simulink model "Vehicle_Model_contABS"  (R2022b)
settings: Solver=ode2  StartTime=T0  StopTime=Tf  FixedStep=Ts  EnableMultiTasking=on
model workspace (MAT data in the model file):
  aKalman = Simulink.Parameter
  aKalman.DataType = 'auto'
  aKalman.Complexity = 'real'
  aKalman.Dimensions = [0 0]
  slipEnabler = Simulink.Parameter
  slipEnabler.DataType = 'auto'
  slipEnabler.Complexity = 'real'
  slipEnabler.Dimensions = [0 0]
values from neighbouring files (symbols this model uses):
  enable_onlinePlots = 0    [main.m]
  enable_zoom = 1    [main.m]
  hv = 0.2    [main.m]
  lambda1_th = 0.1    [main.m]
  lambda2_th = 0.1    [main.m]
  LLC_sampleTime = LLC.sample_time    [main.m]
  longCTRparam = longitController()    [main.m]
  low_level_control = scenario_data.vehicle_control.low_level_control    [main.m]
  omega_LPF = 100    [main.m]
  previewPointParams = previewPointControllerParams()    [main.m]
  rho = 0.97    [main.m]
  rho_off = 0.9    [main.m]
  rho_on = 1.02    [main.m]
  road_data_sampled = [scenario_data.path.x_sampled', scenario_data.path.y_sampled']    [main.m]
  T0 = scenario_data.times.t0    [main.m]
  tau_delta = vehicle_data.steering_system.tau_D    [main.m]
  Tb_dot_max = 5e3    (= 5000)    [main.m]
  Tb_max = 3500    [main.m]
  Tf = scenario_data.times.tf    [main.m]
  Ts = scenario_data.times.step_size    [main.m]
  v_on = 2.5    [main.m]
  v_stop = 0.1    [main.m]
  vehicle_data = getVehicleDataStruct()    [main.m]
  X0 = loadInitialConditions(scenario_data.vehicle_control.max_speed/3.6)    [main.m]
undefined symbols (not defined in the file or in its folder): DiscIntNeverNeededParam, latContr_select
libraries: simulink_extras x20, simulink x9, dspsigops x4, drivingvehiclecontroller x2
(part 1 of 2)
settings Model: Creator=Edoardo  LastModifiedBy=giacomo
settings SolverCC: AlgebraicLoopSolver=TrustRegion
settings DataIOCC: LimitDataPoints=on  SaveFormat=Array
settings OptimizationCC: DefaultParameterBehavior=Inlined  PassReuseOutputArgsAs=Individual arguments  MaxStackSize=64  EfficientTunableParamExpr=on
settings DebuggingCC: ReadBeforeWriteMsg=DisableAll  WriteAfterWriteMsg=DisableAll  WriteAfterReadMsg=DisableAll  MultiTaskDSMMsg=none  ParameterTunabilityLossMsg=error  UnconnectedInputMsg=warning  UnconnectedOutputMsg=warning  UnconnectedLineMsg=warning  PregeneratedLibrarySubsystemCodeDiagnostic=none  SFUnexpectedBacktrackingDiag=warning  SFNoUnconditionalDefaultTransitionDiag=warning  SFExecutionAtInitializationDiag=none  SFMachineParentedDataDiag=warning  ArithmeticOperatorsInVariantConditions=warning
settings HardwareCC: ProdBitPerInt=16  ProdBitPerPointer=16  ProdBitPerSizeT=16  ProdBitPerPtrDiffT=16  ProdLargestAtomicFloat=None  ProdWordSize=16  ProdHWDeviceType=STMicroelectronics->ST10/Super10
settings ModelReferenceCC: UpdateModelReferenceTargets=IfOutOfDate  EnableRefExpFcnMdlSchedulingChecks=on  PropagateSignalLabelsOutOfModel=off
settings SFSimCC: SFSimEcho=off  SimUseLocalCustomCode=off  MATLABDynamicMemAlloc=off  CustomCodeUndefinedFunction=UseInterfaceOnly
settings RTWCC: Description=Embedded Coder  SystemTargetFile=ert.tlc  TemplateMakefile=ert_default_tmf  GenerateReport=on  RetainRTWFile=on  RTWUseLocalCustomCode=off  Toolchain=GNU Tools for ARM Embedded Processors  BuildConfiguration=Faster Runs  IncludeHyperlinkInReport=on  LaunchReport=on  GenerateTraceInfo=on  GenerateTraceReport=on  GenerateTraceReportSl=on  GenerateTraceReportSf=on  GenerateTraceReportEml=on  DLArmComputeVersion=19.05
settings CodeAppCC: ForceParamTrailComments=on  IgnoreCustomStorageClasses=off  OperatorAnnotations=on  SimulinkDataObjDesc=on  SFDataObjDesc=on  InsertBlockDesc=on
settings ERTTargetCC: CodeReplacementLibrary=ARM Cortex-M (Optimized)  SupportVariableSizeSignals=on  RootIOFormat=Structure reference  ERTCustomFileTemplate=example_file_process.tlc
settings ConfigComp: CovMetricSettings=dw  CovSaveCumulativeToWorkspaceVar=on  CovSaveSingleToWorkspaceVar=on  CovExternalEMLEnable=off

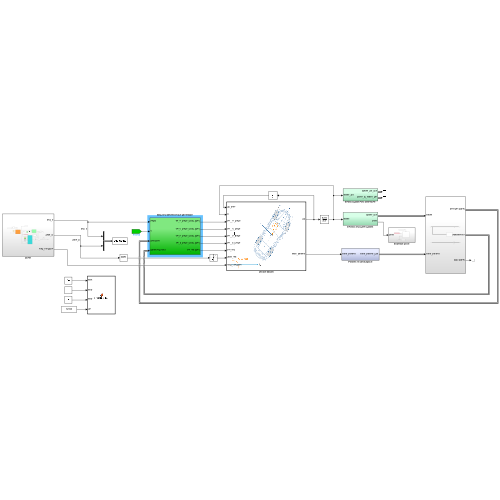
[thumbnail: Simulink's stored preview of the top-level diagram]
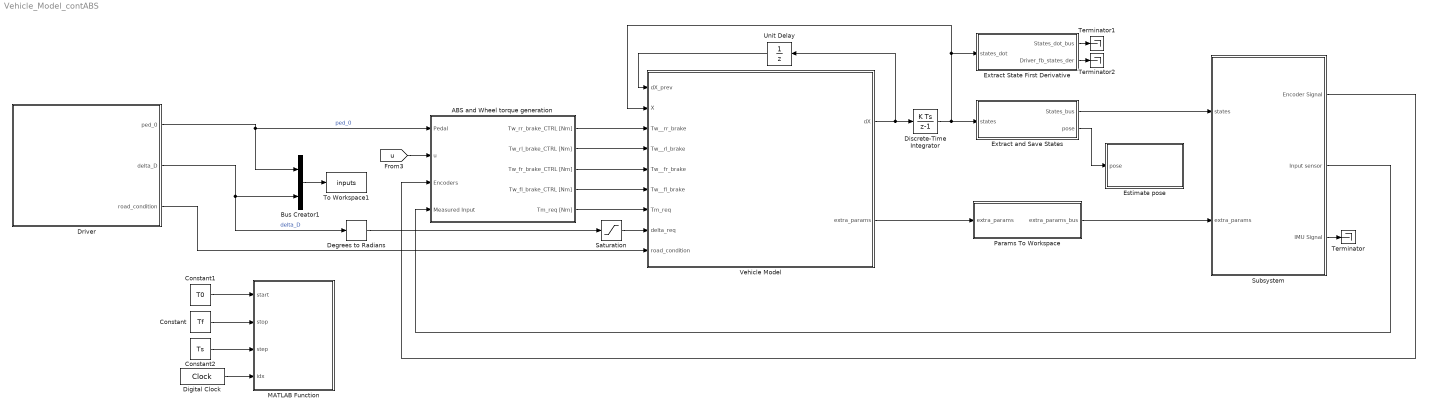
== system Vehicle_Model_contABS ==
  ABS and Wheel torque generation : Subsystem
  Bus Creator1 : BusCreator  Inputs=2
  Constant : Constant  Value=Tf
  Constant1 : Constant  Value=T0
  Constant2 : Constant  Value=Ts
  Degrees to Radians : simulink_extras/Transformations/Degrees to Radians
  Digital Clock : DigitalClock
  Discrete-Time Integrator : DiscreteIntegrator  gainval=1  InitialCondition=X0  SampleTime=-1  ICPrevOutput=DiscIntNeverNeededParam  ICPrevScaledInput=DiscIntNeverNeededParam
  Driver : Subsystem
  Estimate pose : Subsystem
  Extract State First Derivative : Subsystem
  Extract and Save States : Subsystem
  MATLAB Function : MATLAB Function  TreatAsAtomicUnit=on
  Params To Workspace : Subsystem
  Saturation : Saturate  UpperLimit=7  LowerLimit=-7
  Subsystem : Subsystem
  Terminator : Terminator
  Terminator1 : Terminator
  Terminator2 : Terminator
  To Workspace1 : ToWorkspace  VariableName=inputs  SaveFormat=Timeseries  SampleTime=-1
  Unit Delay : UnitDelay  InitialCondition=zeros(size(X0))  SampleTime=-1  HasFrameUpgradeWarning=on
  Vehicle Model : MATLAB Function  TreatAsAtomicUnit=on
  wires:
  ABS and Wheel torque generation/1(Tw_rr_brake_CTRL [Nm]) -> Vehicle Model/3(Tw__rr_brake)
  Subsystem/2(Input sensor) -> ABS and Wheel torque generation/4(Measured Input)
  Degrees to Radians/1 -> Saturation/1
  Bus Creator1/1 -> To Workspace1/1
  Extract and Save States/1(States_bus) -> Subsystem/1(states)
  ABS and Wheel torque generation/3(Tw_fr_brake_CTRL [Nm]) -> Vehicle Model/5(Tw__fr_brake)
  Vehicle Model/1(dX) -> Unit Delay/1, Discrete-Time Integrator/1
  Extract State First Derivative/2(Driver_fb_states_der) -> Terminator2/1
  Subsystem/1(Encoder Signal) -> ABS and Wheel torque generation/3(Encoders)
  Unit Delay/1 -> Vehicle Model/1(dX_prev)
  Extract State First Derivative/1(States_dot_bus) -> Terminator1/1
  Driver/2(delta_D) -> Degrees to Radians/1, Bus Creator1/2  "delta_D"
  Discrete-Time Integrator/1 -> Extract and Save States/1(states), Extract State First Derivative/1(states_dot), Vehicle Model/2(X)
  Vehicle Model/2(extra_params) -> Params To Workspace/1(extra_params)
  ABS and Wheel torque generation/2(Tw_rl_brake_CTRL [Nm]) -> Vehicle Model/4(Tw__rl_brake)
  ABS and Wheel torque generation/5(Tm_req [Nm]) -> Vehicle Model/7(Tm_req)
  Driver/1(ped_0) -> Bus Creator1/1, ABS and Wheel torque generation/1(Pedal)  "ped_0"
  ABS and Wheel torque generation/4(Tw_fl_brake_CTRL [Nm]) -> Vehicle Model/6(Tw__fl_brake)
  Params To Workspace/1(extra_params_bus) -> Subsystem/2(extra_params)
  Constant/1 -> MATLAB Function/2(stop)
  Constant1/1 -> MATLAB Function/1(start)
  Digital Clock/1 -> MATLAB Function/4(idx)
  Constant2/1 -> MATLAB Function/3(step)
  Extract and Save States/2(pose) -> Estimate pose/1(pose)
  [u] -> ABS and Wheel torque generation/2(u)
  Saturation/1 -> Vehicle Model/8(delta_req)
  Driver/3(road_condition) -> Vehicle Model/9(road_condition)
  Subsystem/3(IMU Signal) -> Terminator/1

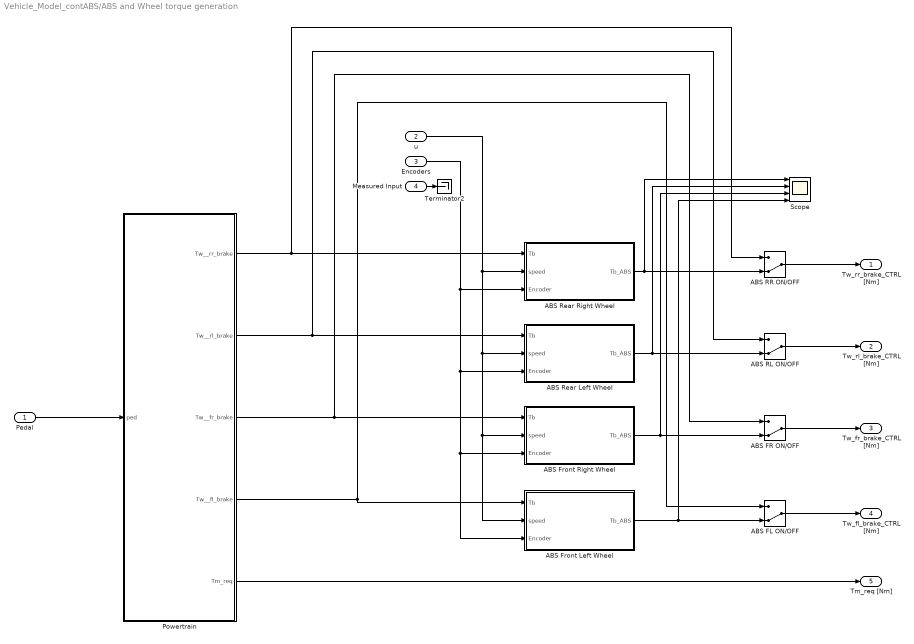
== system Vehicle_Model_contABS/ABS and Wheel torque generation ==
  Pedal : Inport
  u : Inport  Port=2
  Encoders : Inport  Port=3
  Measured Input : Inport  Port=4
  ABS FL ON/OFF : ManualSwitch  CurrentSetting=0
  ABS FR ON/OFF : ManualSwitch  CurrentSetting=0
  ABS Front Left Wheel : Subsystem
  ABS Front Right Wheel : Subsystem
  ABS RL ON/OFF : ManualSwitch  CurrentSetting=0
  ABS RR ON/OFF : ManualSwitch  CurrentSetting=0
  ABS Rear Left Wheel : Subsystem
  ABS Rear Right Wheel : Subsystem
  Powertrain : MATLAB Function  TreatAsAtomicUnit=on
  Scope : Scope  NumInputPorts=4
  Terminator2 : Terminator
  Tw_rr_brake_CTRL [Nm] : Outport  VectorParamsAs1DForOutWhenUnconnected=off
  Tw_rl_brake_CTRL [Nm] : Outport  Port=2  VectorParamsAs1DForOutWhenUnconnected=off
  Tw_fr_brake_CTRL [Nm] : Outport  Port=3  VectorParamsAs1DForOutWhenUnconnected=off
  Tw_fl_brake_CTRL [Nm] : Outport  Port=4  VectorParamsAs1DForOutWhenUnconnected=off
  Tm_req [Nm] : Outport  Port=5  VectorParamsAs1DForOutWhenUnconnected=off
  wires:
  Powertrain/3(Tw__fr_brake) -> ABS FR ON/OFF/1, ABS Front Right Wheel/1(Tb)
  ABS FL ON/OFF/1 -> Tw_fl_brake_CTRL [Nm]/1
  Powertrain/5(Tm_req) -> Tm_req [Nm]/1
  ABS FR ON/OFF/1 -> Tw_fr_brake_CTRL [Nm]/1
  u/1 -> ABS Rear Right Wheel/2(speed), ABS Front Left Wheel/2(speed), ABS Front Right Wheel/2(speed), ABS Rear Left Wheel/2(speed)
  ABS RL ON/OFF/1 -> Tw_rl_brake_CTRL [Nm]/1
  Powertrain/2(Tw__rl_brake) -> ABS RL ON/OFF/1, ABS Rear Left Wheel/1(Tb)
  Pedal/1 -> Powertrain/1(ped)
  ABS RR ON/OFF/1 -> Tw_rr_brake_CTRL [Nm]/1
  Encoders/1 -> ABS Rear Right Wheel/3(Encoder), ABS Rear Left Wheel/3(Encoder), ABS Front Right Wheel/3(Encoder), ABS Front Left Wheel/3(Encoder)
  Measured Input/1 -> Terminator2/1
  Powertrain/4(Tw__fl_brake) -> ABS Front Left Wheel/1(Tb), ABS FL ON/OFF/1
  ABS Rear Left Wheel/1(Tb_ABS) -> Scope/2, ABS RL ON/OFF/2
  ABS Front Right Wheel/1(Tb_ABS) -> Scope/3, ABS FR ON/OFF/2
  ABS Front Left Wheel/1(Tb_ABS) -> Scope/4, ABS FL ON/OFF/2
  ABS Rear Right Wheel/1(Tb_ABS) -> Scope/1, ABS RR ON/OFF/2
  Powertrain/1(Tw__rr_brake) -> ABS Rear Right Wheel/1(Tb), ABS RR ON/OFF/1

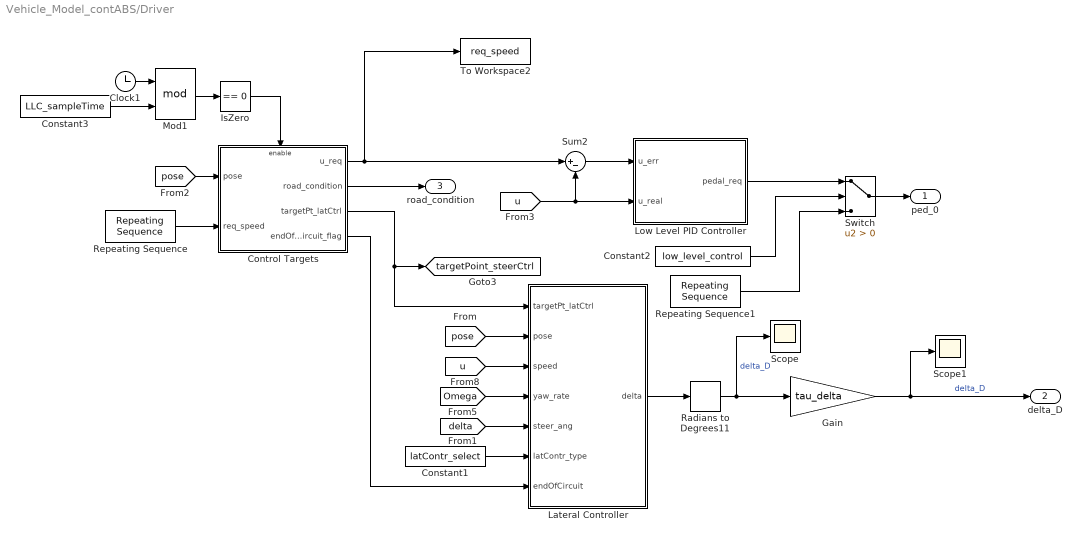
== system Vehicle_Model_contABS/Driver ==
  Clock1 : Clock
  Constant1 : Constant  Value=latContr_select
  Constant2 : Constant  Value=low_level_control
  Constant3 : Constant  Value=LLC_sampleTime
  Control Targets : Subsystem
  Gain : Gain  Gain=tau_delta
  IsZero : simulink/Logic and Bit Operations/Compare To Zero  relop===  OutDataTypeStr=boolean
  Lateral Controller : Subsystem
  Low Level PID Controller : Subsystem
  Mod1 : Math  Operator=mod  SignedPower=on
  Radians to Degrees11 : simulink_extras/Transformations/Radians to Degrees
  Repeating Sequence : simulink/Sources/Repeating Sequence  rep_seq_t=time_manoeuvre  rep_seq_y=req_speed
  Repeating Sequence1 : simulink/Sources/Repeating Sequence  rep_seq_t=time_pedal  rep_seq_y=req_pedal
  Scope : Scope
  Scope1 : Scope
  Sum2 : Sum  Inputs=|+-
  Switch : Switch  Criteria=u2 > Threshold  SaturateOnIntegerOverflow=off  InputSameDT=off
  To Workspace2 : ToWorkspace  VariableName=req_speed  SaveFormat=Timeseries  SampleTime=-1
  ped_0 : Outport  PortDimensions=1
  delta_D : Outport  Port=2  PortDimensions=1
  road_condition : Outport  Port=3
  tag scope: targetPoint_steerCtrl=global
  wires:
  Constant1/1 -> Lateral Controller/6(latContr_type)
  [pose] -> Lateral Controller/2(pose)
  [pose] -> Control Targets/1(pose)
  IsZero/1 -> Control Targets/Enable
  [u] -> Lateral Controller/3(speed)
  [u] -> Sum2/2, Low Level PID Controller/2(u_real)
  Clock1/1 -> Mod1/1
  Control Targets/1(u_req) -> Sum2/1, To Workspace2/1
  [Omega] -> Lateral Controller/4(yaw_rate)
  Sum2/1 -> Low Level PID Controller/1(u_err)
  Constant3/1 -> Mod1/2
  Mod1/1 -> IsZero/1
  Control Targets/3(targetPt_latCtrl) -> Lateral Controller/1(targetPt_latCtrl), [targetPoint_steerCtrl]
  [delta] -> Lateral Controller/5(steer_ang)
  Lateral Controller/1(delta) -> Radians to Degrees11/1
  Control Targets/4(endOfCircuit_flag) -> Lateral Controller/7(endOfCircuit)
  Gain/1 -> Scope1/1, delta_D/1  "delta_D"
  Repeating Sequence/1 -> Control Targets/2(req_speed)
  Switch/1 -> ped_0/1
  Repeating Sequence1/1 -> Switch/3
  Low Level PID Controller/1(pedal_req) -> Switch/1
  Radians to Degrees11/1 -> Gain/1, Scope/1  "delta_D"
  Control Targets/2(road_condition) -> road_condition/1
  Constant2/1 -> Switch/2

== system Vehicle_Model_contABS/Estimate pose ==
  pose : Inport
  Constant3 : Constant  Value=enable_onlinePlots
  Online Trajectory Plots : Subsystem
      mask Display: image('example_path.png'); % Use "Edit Image" on toolstrip to change.
  To Workspace4 : ToWorkspace  VariableName=vehicle_pose  SampleTime=-1
      settings: Save2DSignal=2-D array (concatenate along first dimension)
  wires:
  [targetPoint_steerCtrl] -> Online Trajectory Plots/1(targetPoint_steerCtrl)
  Constant3/1 -> Online Trajectory Plots/Enable
  pose/1 -> To Workspace4/1, Online Trajectory Plots/2(pose)

== system Vehicle_Model_contABS/Extract State First Derivative ==
  states_dot : Inport
  Bus Creator1 : BusCreator  Inputs=23
  Bus Selector : BusSelector  OutputSignals=Omega,x,y,u  OutputAsBus=on
  Demux1 : Demux  Outputs=23
  Radians to Degrees{1..4} (4 alike) : simulink_extras/Transformations/Radians to Degrees
  States_dot_bus : Outport
  Driver_fb_states_der : Outport  Port=2
  wires:
  Demux1/13 -> Bus Creator1/13  "omega_rl"
  Demux1/8 -> Bus Creator1/8  "Fz_rl"
  Demux1/23 -> Bus Creator1/23  "kappa_fl"
  Demux1/19 -> Radians to Degrees4/1
  states_dot/1 -> Demux1/1
  Demux1/14 -> Bus Creator1/14  "omega_fr"
  Demux1/7 -> Bus Creator1/7  "Fz_rr"
  Demux1/15 -> Bus Creator1/15  "omega_fl"
  Demux1/3 -> Bus Creator1/3  "psi"
  Demux1/22 -> Bus Creator1/22  "kappa_fr"
  Demux1/4 -> Bus Creator1/4  "u"
  Demux1/6 -> Bus Creator1/6  "Omega"
  Demux1/11 -> Bus Creator1/11  "delta"
  Demux1/5 -> Bus Creator1/5  "v"
  Demux1/9 -> Bus Creator1/9  "Fz_fr"
  Demux1/21 -> Bus Creator1/21  "kappa_rl"
  Demux1/12 -> Bus Creator1/12  "omega_rr"
  Demux1/17 -> Radians to Degrees1/1
  Demux1/2 -> Bus Creator1/2  "y"
  Demux1/20 -> Bus Creator1/20  "kappa_rr"
  Demux1/10 -> Bus Creator1/10  "Fz_fl"
  Demux1/18 -> Radians to Degrees3/1
  Demux1/1 -> Bus Creator1/1  "x"
  Demux1/16 -> Radians to Degrees2/1
  Bus Creator1/1 -> Bus Selector/1, States_dot_bus/1
  Radians to Degrees2/1 -> Bus Creator1/16  "alpha_rr"
  Radians to Degrees1/1 -> Bus Creator1/17  "alpha_rl"
  Radians to Degrees3/1 -> Bus Creator1/18  "alpha_fr"
  Radians to Degrees4/1 -> Bus Creator1/19  "alpha_fl"
  Bus Selector/1 -> Driver_fb_states_der/1

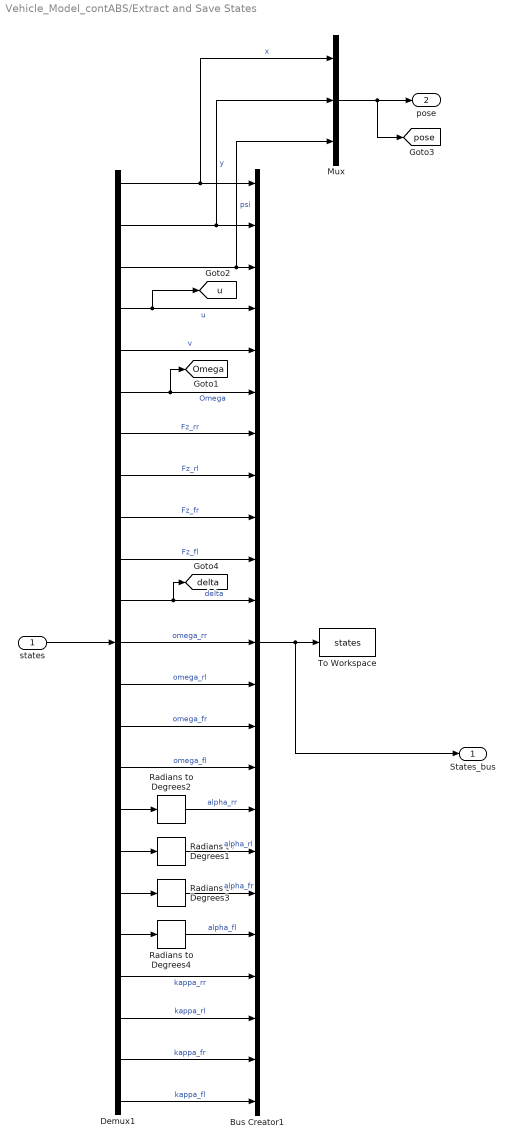
== system Vehicle_Model_contABS/Extract and Save States ==
  states : Inport
  Bus Creator1 : BusCreator  Inputs=23
  Demux1 : Demux  Outputs=23
  Mux : Mux  Inputs=3
  Radians to Degrees{1..4} (4 alike) : simulink_extras/Transformations/Radians to Degrees
  To Workspace : ToWorkspace  VariableName=states  SaveFormat=Timeseries  SampleTime=-1
  States_bus : Outport
  pose : Outport  Port=2
  tag scope: Omega=global, delta=global, pose=global, u=global
  wires:
  Demux1/13 -> Bus Creator1/13  "omega_rl"
  Demux1/8 -> Bus Creator1/8  "Fz_rl"
  Demux1/23 -> Bus Creator1/23  "kappa_fl"
  Demux1/19 -> Radians to Degrees4/1
  states/1 -> Demux1/1
  Demux1/14 -> Bus Creator1/14  "omega_fr"
  Demux1/7 -> Bus Creator1/7  "Fz_rr"
  Demux1/15 -> Bus Creator1/15  "omega_fl"
  Demux1/22 -> Bus Creator1/22  "kappa_fr"
  Demux1/6 -> [Omega], Bus Creator1/6  "Omega"
  Demux1/11 -> [delta], Bus Creator1/11  "delta"
  Demux1/5 -> Bus Creator1/5  "v"
  Demux1/9 -> Bus Creator1/9  "Fz_fr"
  Demux1/21 -> Bus Creator1/21  "kappa_rl"
  Demux1/12 -> Bus Creator1/12  "omega_rr"
  Demux1/17 -> Radians to Degrees1/1
  Demux1/20 -> Bus Creator1/20  "kappa_rr"
  Demux1/10 -> Bus Creator1/10  "Fz_fl"
  Demux1/18 -> Radians to Degrees3/1
  Demux1/16 -> Radians to Degrees2/1
  Bus Creator1/1 -> States_bus/1, To Workspace/1
  Radians to Degrees2/1 -> Bus Creator1/16  "alpha_rr"
  Radians to Degrees1/1 -> Bus Creator1/17  "alpha_rl"
  Radians to Degrees3/1 -> Bus Creator1/18  "alpha_fr"
  Radians to Degrees4/1 -> Bus Creator1/19  "alpha_fl"
  Demux1/1 -> Mux/1, Bus Creator1/1  "x"
  Demux1/3 -> Mux/3, Bus Creator1/3  "psi"
  Demux1/4 -> [u], Bus Creator1/4  "u"
  Demux1/2 -> Bus Creator1/2, Mux/2  "y"
  Mux/1 -> [pose], pose/1

== system Vehicle_Model_contABS/Params To Workspace ==
  extra_params : Inport
  Bus Creator2 : BusCreator  Inputs=23
  Demux1 : Demux  Outputs=23
  Radians to Degrees{,1..4,11..12} (7 alike) : simulink_extras/Transformations/Radians to Degrees
  To Workspace2 : ToWorkspace  VariableName=extra_params  SaveFormat=Timeseries  SampleTime=-1
  extra_params_bus : Outport
  wires:
  Demux1/17 -> Radians to Degrees1/1
  Demux1/3 -> Bus Creator2/3  "Tw_fr"
  Radians to Degrees3/1 -> Bus Creator2/20  "gamma_fl"
  Demux1/16 -> Bus Creator2/16  "Mz_fl"
  Radians to Degrees1/1 -> Bus Creator2/17  "gamma_rr"
  Radians to Degrees11/1 -> Bus Creator2/21  "delta_fr"
  Demux1/14 -> Bus Creator2/14  "Mz_rl"
  Demux1/4 -> Bus Creator2/4  "Tw_fl"
  Demux1/6 -> Bus Creator2/6  "Fx_rl"
  Demux1/8 -> Bus Creator2/8  "Fx_fl"
  Demux1/13 -> Bus Creator2/13  "Mz_rr"
  Demux1/7 -> Bus Creator2/7  "Fx_fr"
  Demux1/5 -> Bus Creator2/5  "Fx_rr"
  Demux1/9 -> Bus Creator2/9  "Fy_rr"
  Demux1/11 -> Bus Creator2/11  "Fy_fr"
  Demux1/15 -> Bus Creator2/15  "Mz_fr"
  Demux1/10 -> Bus Creator2/10  "Fy_rl"
  Radians to Degrees12/1 -> Bus Creator2/22  "delta_fl"
  Radians to Degrees2/1 -> Bus Creator2/19  "gamma_fr"
  extra_params/1 -> Demux1/1
  Demux1/12 -> Bus Creator2/12  "Fy_fl"
  Bus Creator2/1 -> To Workspace2/1, extra_params_bus/1
  Demux1/1 -> Bus Creator2/1  "Tw_rr"
  Demux1/2 -> Bus Creator2/2  "Tw_rl"
  Radians to Degrees/1 -> Bus Creator2/18  "gamma_rl"
  Demux1/18 -> Radians to Degrees/1
  Demux1/19 -> Radians to Degrees2/1
  Demux1/20 -> Radians to Degrees3/1
  Demux1/21 -> Radians to Degrees11/1
  Demux1/22 -> Radians to Degrees12/1
  Demux1/23 -> Radians to Degrees4/1
  Radians to Degrees4/1 -> Bus Creator2/23  "delta_SW"

== system Vehicle_Model_contABS/Subsystem ==
  states : Inport
  extra_params : Inport  Port=2
  Bus Selector : BusSelector  OutputSignals=omega_rr,omega_rl,omega_fr,omega_fl  OutputAsBus=on
  Bus Selector1 : BusSelector  OutputSignals=delta_SW,Tw_rr,Tw_rl,Tw_fr,Tw_fl  OutputAsBus=on
  IMU : Subsystem
  Encoder Signal : Outport  VectorParamsAs1DForOutWhenUnconnected=off
  Input sensor : Outport  Port=2  VectorParamsAs1DForOutWhenUnconnected=off
  IMU Signal : Outport  Port=3  VectorParamsAs1DForOutWhenUnconnected=off
  wires:
  states/1 -> IMU/1(states), Bus Selector/1
  Bus Selector/1 -> Encoder Signal/1
  IMU/1(IMU) -> IMU Signal/1
  extra_params/1 -> Bus Selector1/1
  Bus Selector1/1 -> Input sensor/1

== system Vehicle_Model_contABS/ABS and Wheel torque generation/ABS Front Left Wheel ==
  Tb : Inport
  speed : Inport  Port=2
  Encoder : Inport  Port=3
  Antilock Braking System : Subsystem
      mask Display: image('ABS_on.png'); % Use "Edit Image" on toolstrip to change.
  Bus Selector : BusSelector  OutputSignals=omega_fl
  Constant : Constant  Value=0.14
  Gain : Gain  Gain=-1
  Gain1 : Gain  Gain=-1
  To Workspace3 : ToWorkspace  VariableName=TwrflCtrl  SaveFormat=Timeseries  SampleTime=-1
  compute lambda : MATLAB Function  TreatAsAtomicUnit=on
  Tb_ABS : Outport  VectorParamsAs1DForOutWhenUnconnected=off
  wires:
  Tb/1 -> Gain/1
  speed/1 -> Antilock Braking System/4(vehicle speed [m/s]), compute lambda/1(u)
  Gain/1 -> Antilock Braking System/1(Tb_Dr [Nm])
  Encoder/1 -> Bus Selector/1
  Antilock Braking System/1(Tb [Nm]) -> Gain1/1
  compute lambda/1(lambda) -> Antilock Braking System/3(lambda [-])
  Bus Selector/1 -> compute lambda/2(omega)  "<omega_fl>"
  Constant/1 -> Antilock Braking System/2(lambda_ref [-])
  Gain1/1 -> Tb_ABS/1, To Workspace3/1

== system Vehicle_Model_contABS/ABS and Wheel torque generation/ABS Front Right Wheel ==
  Tb : Inport
  speed : Inport  Port=2
  Encoder : Inport  Port=3
  Antilock Braking System : Subsystem
      mask Display: image('ABS_on.png'); % Use "Edit Image" on toolstrip to change.
  Bus Selector : BusSelector  OutputSignals=omega_fr
  Constant : Constant  Value=0.14
  Gain : Gain  Gain=-1
  Gain1 : Gain  Gain=-1
  To Workspace3 : ToWorkspace  VariableName=TwfrCtrl  SaveFormat=Timeseries  SampleTime=-1
  compute lambda : MATLAB Function  TreatAsAtomicUnit=on
  Tb_ABS : Outport  VectorParamsAs1DForOutWhenUnconnected=off
  wires:
  Tb/1 -> Gain/1
  speed/1 -> Antilock Braking System/4(vehicle speed [m/s]), compute lambda/1(u)
  Gain/1 -> Antilock Braking System/1(Tb_Dr [Nm])
  Encoder/1 -> Bus Selector/1
  Antilock Braking System/1(Tb [Nm]) -> Gain1/1
  compute lambda/1(lambda) -> Antilock Braking System/3(lambda [-])
  Bus Selector/1 -> compute lambda/2(omega)  "<omega_fr>"
  Constant/1 -> Antilock Braking System/2(lambda_ref [-])
  Gain1/1 -> To Workspace3/1, Tb_ABS/1

== system Vehicle_Model_contABS/ABS and Wheel torque generation/ABS Rear Left Wheel ==
  Tb : Inport
  speed : Inport  Port=2
  Encoder : Inport  Port=3
  Antilock Braking System : Subsystem
      mask Display: image('ABS_on.png'); % Use "Edit Image" on toolstrip to change.
  Bus Selector : BusSelector  OutputSignals=omega_rl
  Constant : Constant  Value=0.14
  Gain : Gain  Gain=-1
  Gain1 : Gain  Gain=-1
  To Workspace3 : ToWorkspace  VariableName=TwrlCtrl  SaveFormat=Timeseries  SampleTime=-1
  compute lambda : MATLAB Function  TreatAsAtomicUnit=on
  Tb_ABS : Outport  VectorParamsAs1DForOutWhenUnconnected=off
  wires:
  Tb/1 -> Gain/1
  speed/1 -> Antilock Braking System/4(vehicle speed [m/s]), compute lambda/1(u)
  Gain/1 -> Antilock Braking System/1(Tb_Dr [Nm])
  Encoder/1 -> Bus Selector/1
  Antilock Braking System/1(Tb [Nm]) -> Gain1/1
  compute lambda/1(lambda) -> Antilock Braking System/3(lambda [-])
  Bus Selector/1 -> compute lambda/2(omega)  "<omega_rl>"
  Constant/1 -> Antilock Braking System/2(lambda_ref [-])
  Gain1/1 -> To Workspace3/1, Tb_ABS/1

== system Vehicle_Model_contABS/ABS and Wheel torque generation/ABS Rear Right Wheel ==
  Tb : Inport
  speed : Inport  Port=2
  Encoder : Inport  Port=3
  Antilock Braking System : Subsystem
      mask Display: image('ABS_on.png'); % Use "Edit Image" on toolstrip to change.
  Bus Selector : BusSelector  OutputSignals=omega_rr
  Constant : Constant  Value=0.14
  Gain : Gain  Gain=-1
  Gain1 : Gain  Gain=-1
  To Workspace3 : ToWorkspace  VariableName=TwrrCtrl  SaveFormat=Timeseries  SampleTime=-1
  compute lambda : MATLAB Function  TreatAsAtomicUnit=on
  Tb_ABS : Outport  VectorParamsAs1DForOutWhenUnconnected=off
  wires:
  Tb/1 -> Gain/1
  speed/1 -> Antilock Braking System/4(vehicle speed [m/s]), compute lambda/1(u)
  Encoder/1 -> Bus Selector/1
  Bus Selector/1 -> compute lambda/2(omega)  "<omega_rr>"
  Gain/1 -> Antilock Braking System/1(Tb_Dr [Nm])
  Antilock Braking System/1(Tb [Nm]) -> Gain1/1
  compute lambda/1(lambda) -> Antilock Braking System/3(lambda [-])
  Constant/1 -> Antilock Braking System/2(lambda_ref [-])
  Gain1/1 -> Tb_ABS/1, To Workspace3/1

== system Vehicle_Model_contABS/Driver/Control Targets ==
  pose : Inport
  req_speed : Inport  Port=2
  Enable : EnablePort
  MATLAB System : MATLABSystem  System=setControlTargets  lateralController_type=latContr_select  purePursuit_lookAhead=purePursuitParams.lookAhead  clothoidBased_lookAhead=clothoidBasedParams.lookAhead  previewPoint_lookAhead=previewPointParams.lookAhead  refRoute_points=road_data  road_condition=road_condition  Lf=vehicle_data.vehicle.Lf  SimulateUsing=Interpreted execution
      mask Type: setControlTargets
      mask Display:
      | disp('setControlTargets');
      | port_label('input',1,'vehPose');
      | port_label('input',2,'req_speed');
      | port_label('output',1,'targetPoint_latControl');
      | port_label('output',2,'speed_req');
      | port_label('output',3,'road_condition');
      | port_label('output',4,'endOfCircuit');
  u_req : Outport  VectorParamsAs1DForOutWhenUnconnected=off
  road_condition : Outport  Port=2
  targetPt_latCtrl : Outport  Port=3  VectorParamsAs1DForOutWhenUnconnected=off
  endOfCircuit_flag : Outport  Port=4  VectorParamsAs1DForOutWhenUnconnected=off
  wires:
  pose/1 -> MATLAB System/1
  MATLAB System/2 -> u_req/1
  MATLAB System/1 -> targetPt_latCtrl/1
  MATLAB System/4 -> endOfCircuit_flag/1
  req_speed/1 -> MATLAB System/2
  MATLAB System/3 -> road_condition/1

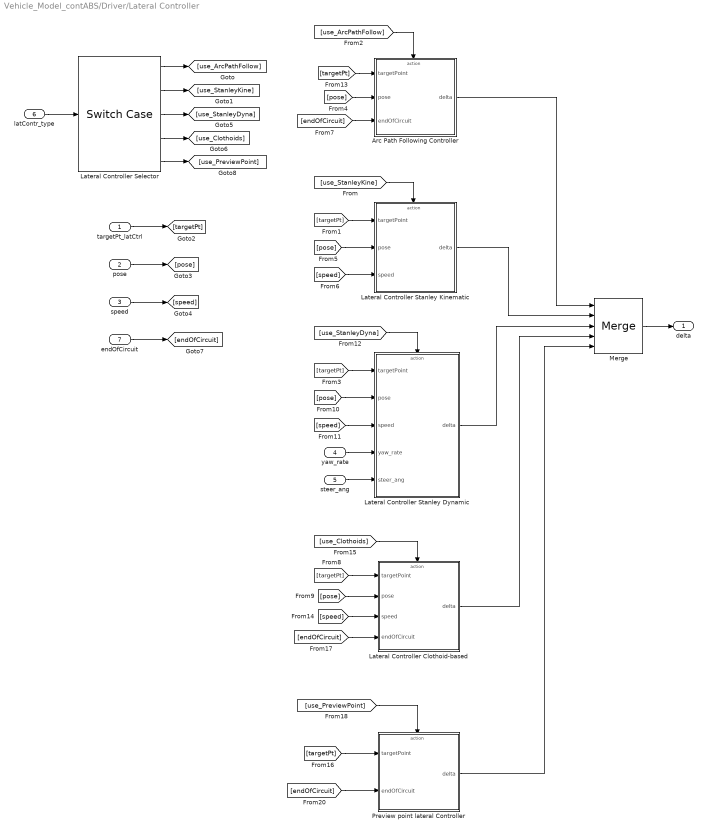
== system Vehicle_Model_contABS/Driver/Lateral Controller ==
  targetPt_latCtrl : Inport
  pose : Inport  Port=2
  speed : Inport  Port=3
  yaw_rate : Inport  Port=4
  steer_ang : Inport  Port=5
  latContr_type : Inport  Port=6
  endOfCircuit : Inport  Port=7
  Arc Path Following Controller : Subsystem  TreatAsAtomicUnit=on
  Lateral Controller Clothoid-based : Subsystem  TreatAsAtomicUnit=on
  Lateral Controller Selector : SwitchCase  CaseConditions={1,2,3,4,5}  ShowDefaultCase=off
  Lateral Controller Stanley Dynamic : Subsystem  TreatAsAtomicUnit=on
  Lateral Controller Stanley Kinematic : Subsystem  TreatAsAtomicUnit=on
  Merge : Merge  Inputs=5
  Preview point lateral Controller : Subsystem  TreatAsAtomicUnit=on
  delta : Outport  VectorParamsAs1DForOutWhenUnconnected=off
  wires:
  Arc Path Following Controller/1(delta) -> Merge/1
  latContr_type/1 -> Lateral Controller Selector/1
  Lateral Controller Stanley Kinematic/1(delta) -> Merge/2
  Merge/1 -> delta/1
  Lateral Controller Selector/1 -> [use_ArcPathFollow]
  [use_ArcPathFollow] -> Arc Path Following Controller/Action
  Lateral Controller Selector/2 -> [use_StanleyKine]
  [use_StanleyKine] -> Lateral Controller Stanley Kinematic/Action
  targetPt_latCtrl/1 -> [targetPt]
  [targetPt] -> Arc Path Following Controller/1(targetPoint)
  [targetPt] -> Lateral Controller Stanley Kinematic/1(targetPoint)
  pose/1 -> [pose]
  [pose] -> Arc Path Following Controller/2(pose)
  [pose] -> Lateral Controller Stanley Kinematic/2(pose)
  speed/1 -> [speed]
  [speed] -> Lateral Controller Stanley Kinematic/3(speed)
  Lateral Controller Selector/3 -> [use_StanleyDyna]
  [pose] -> Lateral Controller Stanley Dynamic/2(pose)
  [targetPt] -> Lateral Controller Stanley Dynamic/1(targetPoint)
  [speed] -> Lateral Controller Stanley Dynamic/3(speed)
  [use_StanleyDyna] -> Lateral Controller Stanley Dynamic/Action
  Lateral Controller Stanley Dynamic/1(delta) -> Merge/3
  yaw_rate/1 -> Lateral Controller Stanley Dynamic/4(yaw_rate)
  steer_ang/1 -> Lateral Controller Stanley Dynamic/5(steer_ang)
  [use_Clothoids] -> Lateral Controller Clothoid-based/Action
  [pose] -> Lateral Controller Clothoid-based/2(pose)
  [targetPt] -> Lateral Controller Clothoid-based/1(targetPoint)
  [speed] -> Lateral Controller Clothoid-based/3(speed)
  Lateral Controller Clothoid-based/1(delta) -> Merge/4
  Lateral Controller Selector/4 -> [use_Clothoids]
  [endOfCircuit] -> Arc Path Following Controller/3(endOfCircuit)
  [endOfCircuit] -> Lateral Controller Clothoid-based/4(endOfCircuit)
  endOfCircuit/1 -> [endOfCircuit]
  [targetPt] -> Preview point lateral Controller/1(targetPoint)
  [endOfCircuit] -> Preview point lateral Controller/2(endOfCircuit)
  [use_PreviewPoint] -> Preview point lateral Controller/Action
  Lateral Controller Selector/5 -> [use_PreviewPoint]
  Preview point lateral Controller/1(delta) -> Merge/5

== system Vehicle_Model_contABS/Driver/Low Level PID Controller ==
  u_err : Inport
  u_real : Inport  Port=2
  1-D Lookup Table : Lookup_n-D  NumberOfTableDimensions=1  BreakpointsForDimension1=longCTRparam.speed_vals_PID_sched  BeginIndexSearchUsingPreviousIndexResult=on  Table=longCTRparam.Kp_vals  ExtrapMethod=Clip  UseLastTableValue=on  InternalRulePriority=Speed  RndMeth=Simplest
  1-D Lookup Table1 : Lookup_n-D  NumberOfTableDimensions=1  BreakpointsForDimension1=longCTRparam.speed_vals_PID_sched  BeginIndexSearchUsingPreviousIndexResult=on  Table=longCTRparam.Ki_vals  ExtrapMethod=Clip  UseLastTableValue=on  InternalRulePriority=Speed  RndMeth=Simplest
  1-D Lookup Table2 : Lookup_n-D  NumberOfTableDimensions=1  BreakpointsForDimension1=longCTRparam.speed_vals_PID_sched  BeginIndexSearchUsingPreviousIndexResult=on  Table=longCTRparam.Kd_vals  ExtrapMethod=Clip  UseLastTableValue=on  InternalRulePriority=Speed  RndMeth=Simplest
  1-D Lookup Table3 : Lookup_n-D  NumberOfTableDimensions=1  BreakpointsForDimension1=longCTRparam.speed_vals_PID_sched  BeginIndexSearchUsingPreviousIndexResult=on  Table=longCTRparam.N_vals  ExtrapMethod=Clip  UseLastTableValue=on  InternalRulePriority=Speed  RndMeth=Simplest
  1-D Lookup Table4 : Lookup_n-D  NumberOfTableDimensions=1  BreakpointsForDimension1=longCTRparam.speed_vals_PID_sched  BeginIndexSearchUsingPreviousIndexResult=on  Table=longCTRparam.Kaw_vals  ExtrapMethod=Clip  UseLastTableValue=on  InternalRulePriority=Speed  RndMeth=Simplest
  Custom Low Level PID : Subsystem
  pedal_req : Outport  VectorParamsAs1DForOutWhenUnconnected=off
  wires:
  1-D Lookup Table/1 -> Custom Low Level PID/2(P)
  u_err/1 -> Custom Low Level PID/1(err)
  u_real/1 -> 1-D Lookup Table4/1, Custom Low Level PID/7(u_veh), 1-D Lookup Table3/1, 1-D Lookup Table2/1, 1-D Lookup Table1/1, 1-D Lookup Table/1
  1-D Lookup Table2/1 -> Custom Low Level PID/4(D)
  1-D Lookup Table3/1 -> Custom Low Level PID/5(N)
  1-D Lookup Table1/1 -> Custom Low Level PID/3(I)
  Custom Low Level PID/1(out_PID) -> pedal_req/1  "pedal_req"
  1-D Lookup Table4/1 -> Custom Low Level PID/6(Kaw)

== system Vehicle_Model_contABS/Estimate pose/Online Trajectory Plots ==
  targetPoint_steerCtrl : Inport
  pose : Inport  Port=2
  Enable : EnablePort
  Constant : Constant  Value=road_data_sampled
  Constant3 : Constant  Value=enable_zoom
  Constant5 : Constant  Value=latContr_select
  Plot manager : MATLAB Function  TreatAsAtomicUnit=on
  wires:
  targetPoint_steerCtrl/1 -> Plot manager/2(targetPoint_steerCtrl)
  Constant/1 -> Plot manager/4(refPath)
  Constant3/1 -> Plot manager/3(enable_zoomMPC)
  pose/1 -> Plot manager/1(vehiclePose)
  Constant5/1 -> Plot manager/5(latContr_type)

== system Vehicle_Model_contABS/Subsystem/IMU ==
  states : Inport
  Bus Creator : BusCreator  Inputs=3
  Bus Selector1 : BusSelector  OutputSignals=u,v,Omega
  Discrete Derivative : simulink/Discrete/Discrete Derivative  gainval=1.0  ICPrevScaledInput=0.0  OutMin=[]  OutMax=[]  OutDataType=fixdt(1, 16)  OutScaling=2^-10  DoSatur=off
  Discrete Derivative1 : simulink/Discrete/Discrete Derivative  gainval=1.0  ICPrevScaledInput=0.0  OutMin=[]  OutMax=[]  OutDataType=fixdt(1, 16)  OutScaling=2^-10  DoSatur=off
  Product : Product
  Product1 : Product
  Sum : Sum  Inputs=+-
  Sum1 : Sum
  IMU : Outport
  wires:
  states/1 -> Bus Selector1/1
  Bus Selector1/1 -> Product1/1, Discrete Derivative/1  "<u>"
  Discrete Derivative/1 -> Sum/1
  Product/1 -> Sum/2
  Bus Selector1/2 -> Discrete Derivative1/1, Product/1  "<v>"
  Bus Selector1/3 -> Product1/2, Bus Creator/3, Product/2  "<Omega>"
  Sum/1 -> Bus Creator/1  "a_x"
  Discrete Derivative1/1 -> Sum1/1
  Product1/1 -> Sum1/2
  Sum1/1 -> Bus Creator/2  "a_y"
  Bus Creator/1 -> IMU/1

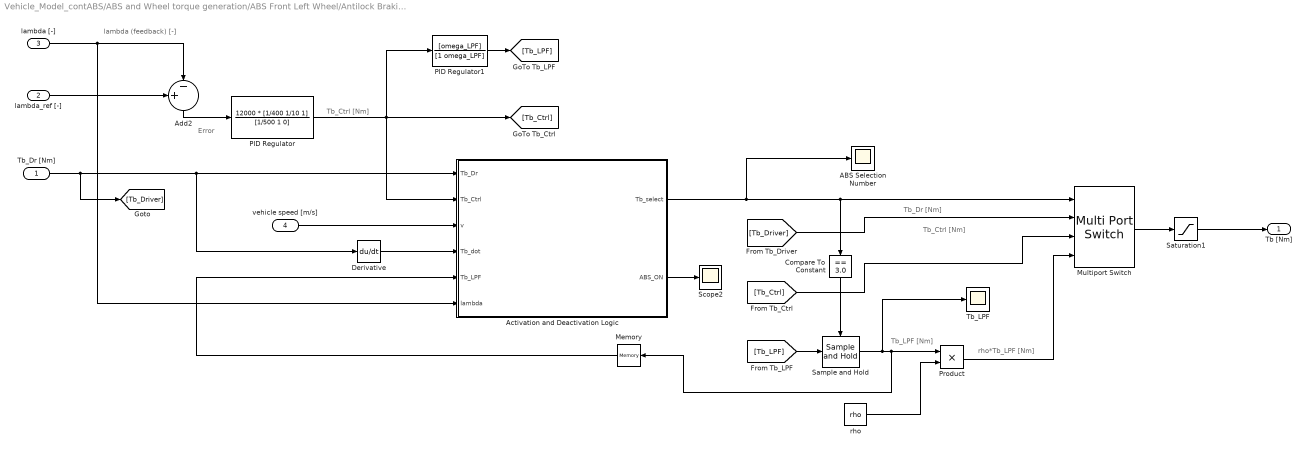
== system Vehicle_Model_contABS/ABS and Wheel torque generation/ABS Front Left Wheel/Antilock Braking System ==
  note: Tb_LPF [Nm]
  note: Tb_Ctrl [Nm]
  note: Tb_Dr [Nm]
  note: lambda (feedback) [-]
  note: Error
  note: Tb_Ctrl [Nm]
  note: rho*Tb_LPF [Nm]
  Tb_Dr [Nm] : Inport
  lambda_ref [-] : Inport  Port=2
  lambda [-] : Inport  Port=3
  vehicle speed [m/s] : Inport  Port=4
  ABS Selection Number : Scope
  Activation and Deactivation Logic : Stateflow chart  TreatAsAtomicUnit=on
  Add2 : Sum  Inputs=+-|
  Compare To Constant : simulink/Logic and Bit Operations/Compare To Constant  relop===  const=3.0  OutDataTypeStr=boolean
  Derivative : Derivative
  Memory : Memory
  Multiport Switch : MultiPortSwitch  SaturateOnIntegerOverflow=off  InputSameDT=off
  PID Regulator : TransferFcn  Numerator=12000 * [1/400 1/10 1]  Denominator=[1/500 1 0]
  PID Regulator1 : TransferFcn  Numerator=[omega_LPF]  Denominator=[1 omega_LPF]
  Product : Product
  Sample and Hold : dspsigops/Sample and Hold  trig=Rising edge  initCond=0  latchinput=off
  Saturation1 : Saturate  UpperLimit=Tb_max  LowerLimit=0
  Scope2 : Scope
  Tb_LPF : Scope
  rho : Constant  Value=rho
  Tb [Nm] : Outport
  wires:
  lambda_ref [-]/1 -> Add2/1
  Activation and Deactivation Logic/2(ABS_ON) -> Scope2/1
  [Tb_Ctrl] -> Multiport Switch/3
  Tb_Dr [Nm]/1 -> [Tb_Driver], Derivative/1, Activation and Deactivation Logic/1(Tb_Dr)
  vehicle speed [m/s]/1 -> Activation and Deactivation Logic/3(v)
  Multiport Switch/1 -> Saturation1/1
  Add2/1 -> PID Regulator/1
  [Tb_Driver] -> Multiport Switch/2
  Derivative/1 -> Activation and Deactivation Logic/4(Tb_dot)
  lambda [-]/1 -> Activation and Deactivation Logic/6(lambda), Add2/2
  Activation and Deactivation Logic/1(Tb_select) -> ABS Selection Number/1, Multiport Switch/1, Compare To Constant/1
  Saturation1/1 -> Tb [Nm]/1
  PID Regulator/1 -> PID Regulator1/1, [Tb_Ctrl], Activation and Deactivation Logic/2(Tb_Ctrl)
  PID Regulator1/1 -> [Tb_LPF]
  [Tb_LPF] -> Sample and Hold/1
  Sample and Hold/1 -> Tb_LPF/1, Product/1, Memory/1
  Memory/1 -> Activation and Deactivation Logic/5(Tb_LPF)
  rho/1 -> Product/2
  Product/1 -> Multiport Switch/4
  Compare To Constant/1 -> Sample and Hold/Trigger

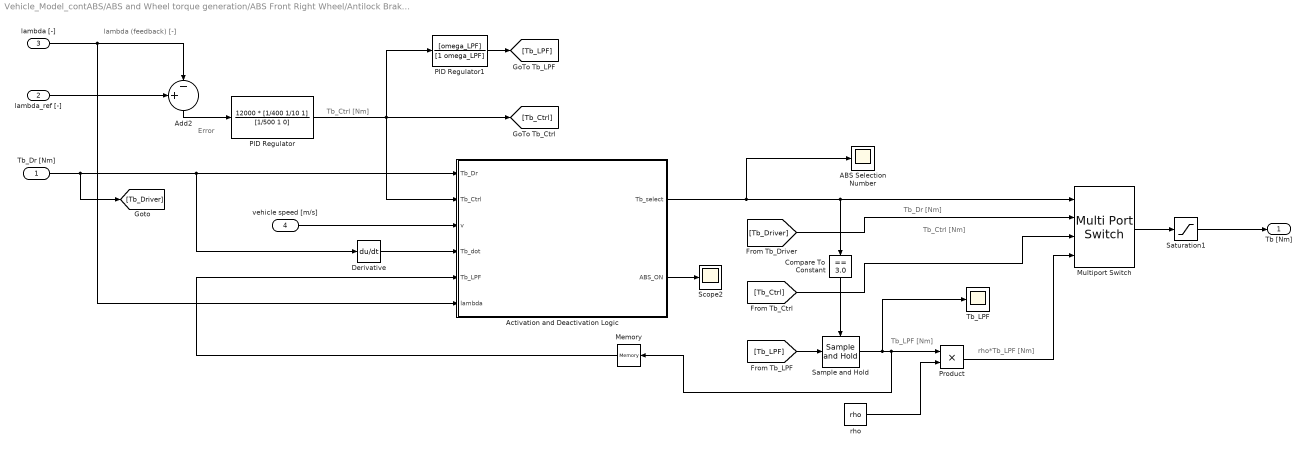
== system Vehicle_Model_contABS/ABS and Wheel torque generation/ABS Front Right Wheel/Antilock Braking System ==
  note: Tb_LPF [Nm]
  note: Tb_Ctrl [Nm]
  note: Tb_Dr [Nm]
  note: lambda (feedback) [-]
  note: Error
  note: Tb_Ctrl [Nm]
  note: rho*Tb_LPF [Nm]
  Tb_Dr [Nm] : Inport
  lambda_ref [-] : Inport  Port=2
  lambda [-] : Inport  Port=3
  vehicle speed [m/s] : Inport  Port=4
  ABS Selection Number : Scope
  Activation and Deactivation Logic : Stateflow chart  TreatAsAtomicUnit=on
  Add2 : Sum  Inputs=+-|
  Compare To Constant : simulink/Logic and Bit Operations/Compare To Constant  relop===  const=3.0  OutDataTypeStr=boolean
  Derivative : Derivative
  Memory : Memory
  Multiport Switch : MultiPortSwitch  SaturateOnIntegerOverflow=off  InputSameDT=off
  PID Regulator : TransferFcn  Numerator=12000 * [1/400 1/10 1]  Denominator=[1/500 1 0]
  PID Regulator1 : TransferFcn  Numerator=[omega_LPF]  Denominator=[1 omega_LPF]
  Product : Product
  Sample and Hold : dspsigops/Sample and Hold  trig=Rising edge  initCond=0  latchinput=off
  Saturation1 : Saturate  UpperLimit=Tb_max  LowerLimit=0
  Scope2 : Scope
  Tb_LPF : Scope
  rho : Constant  Value=rho
  Tb [Nm] : Outport
  wires:
  lambda_ref [-]/1 -> Add2/1
  Activation and Deactivation Logic/2(ABS_ON) -> Scope2/1
  [Tb_Ctrl] -> Multiport Switch/3
  Tb_Dr [Nm]/1 -> [Tb_Driver], Derivative/1, Activation and Deactivation Logic/1(Tb_Dr)
  vehicle speed [m/s]/1 -> Activation and Deactivation Logic/3(v)
  Multiport Switch/1 -> Saturation1/1
  Add2/1 -> PID Regulator/1
  [Tb_Driver] -> Multiport Switch/2
  Derivative/1 -> Activation and Deactivation Logic/4(Tb_dot)
  lambda [-]/1 -> Activation and Deactivation Logic/6(lambda), Add2/2
  Activation and Deactivation Logic/1(Tb_select) -> ABS Selection Number/1, Multiport Switch/1, Compare To Constant/1
  Saturation1/1 -> Tb [Nm]/1
  PID Regulator/1 -> PID Regulator1/1, [Tb_Ctrl], Activation and Deactivation Logic/2(Tb_Ctrl)
  PID Regulator1/1 -> [Tb_LPF]
  [Tb_LPF] -> Sample and Hold/1
  Sample and Hold/1 -> Tb_LPF/1, Product/1, Memory/1
  Memory/1 -> Activation and Deactivation Logic/5(Tb_LPF)
  rho/1 -> Product/2
  Product/1 -> Multiport Switch/4
  Compare To Constant/1 -> Sample and Hold/Trigger

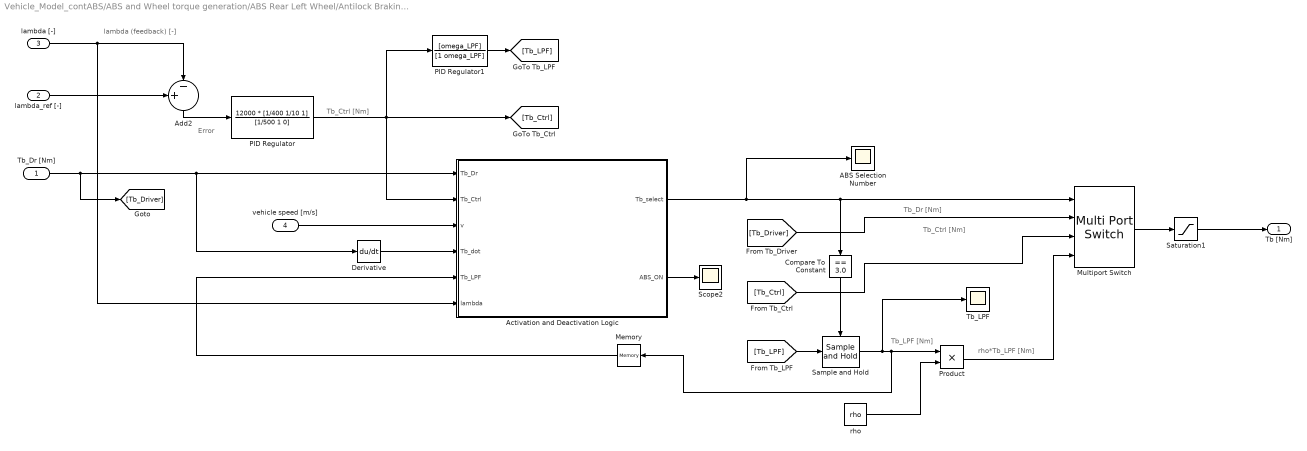
== system Vehicle_Model_contABS/ABS and Wheel torque generation/ABS Rear Left Wheel/Antilock Braking System ==
  note: Tb_LPF [Nm]
  note: Tb_Ctrl [Nm]
  note: Tb_Dr [Nm]
  note: lambda (feedback) [-]
  note: Error
  note: Tb_Ctrl [Nm]
  note: rho*Tb_LPF [Nm]
  Tb_Dr [Nm] : Inport
  lambda_ref [-] : Inport  Port=2
  lambda [-] : Inport  Port=3
  vehicle speed [m/s] : Inport  Port=4
  ABS Selection Number : Scope
  Activation and Deactivation Logic : Stateflow chart  TreatAsAtomicUnit=on
  Add2 : Sum  Inputs=+-|
  Compare To Constant : simulink/Logic and Bit Operations/Compare To Constant  relop===  const=3.0  OutDataTypeStr=boolean
  Derivative : Derivative
  Memory : Memory
  Multiport Switch : MultiPortSwitch  SaturateOnIntegerOverflow=off  InputSameDT=off
  PID Regulator : TransferFcn  Numerator=12000 * [1/400 1/10 1]  Denominator=[1/500 1 0]
  PID Regulator1 : TransferFcn  Numerator=[omega_LPF]  Denominator=[1 omega_LPF]
  Product : Product
  Sample and Hold : dspsigops/Sample and Hold  trig=Rising edge  initCond=0  latchinput=off
  Saturation1 : Saturate  UpperLimit=Tb_max  LowerLimit=0
  Scope2 : Scope
  Tb_LPF : Scope
  rho : Constant  Value=rho
  Tb [Nm] : Outport
  wires:
  lambda_ref [-]/1 -> Add2/1
  Activation and Deactivation Logic/2(ABS_ON) -> Scope2/1
  [Tb_Ctrl] -> Multiport Switch/3
  Tb_Dr [Nm]/1 -> [Tb_Driver], Derivative/1, Activation and Deactivation Logic/1(Tb_Dr)
  vehicle speed [m/s]/1 -> Activation and Deactivation Logic/3(v)
  Multiport Switch/1 -> Saturation1/1
  Add2/1 -> PID Regulator/1
  [Tb_Driver] -> Multiport Switch/2
  Derivative/1 -> Activation and Deactivation Logic/4(Tb_dot)
  lambda [-]/1 -> Activation and Deactivation Logic/6(lambda), Add2/2
  Activation and Deactivation Logic/1(Tb_select) -> ABS Selection Number/1, Multiport Switch/1, Compare To Constant/1
  Saturation1/1 -> Tb [Nm]/1
  PID Regulator/1 -> PID Regulator1/1, [Tb_Ctrl], Activation and Deactivation Logic/2(Tb_Ctrl)
  PID Regulator1/1 -> [Tb_LPF]
  [Tb_LPF] -> Sample and Hold/1
  Sample and Hold/1 -> Tb_LPF/1, Product/1, Memory/1
  Memory/1 -> Activation and Deactivation Logic/5(Tb_LPF)
  rho/1 -> Product/2
  Product/1 -> Multiport Switch/4
  Compare To Constant/1 -> Sample and Hold/Trigger

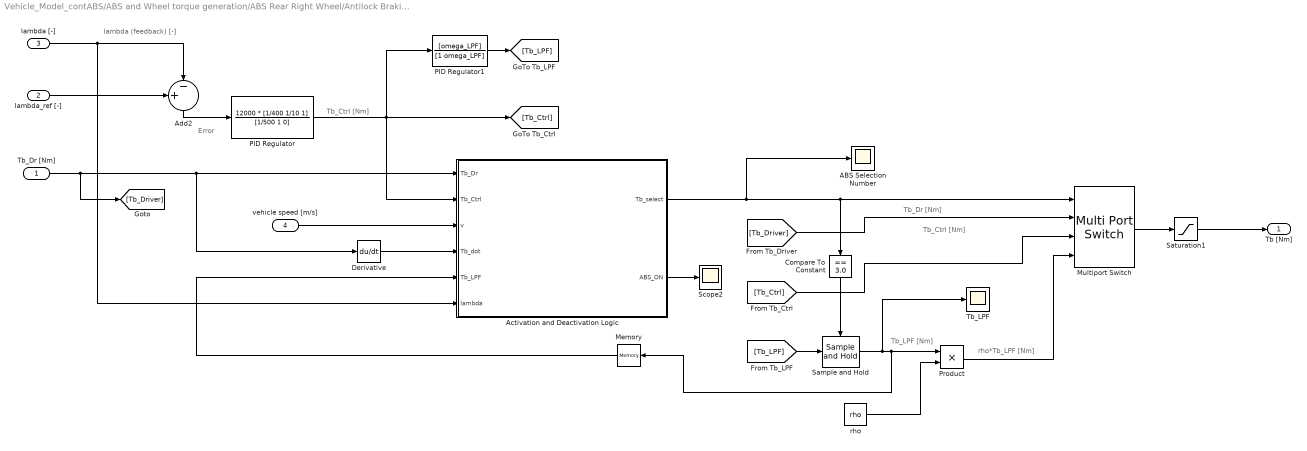
== system Vehicle_Model_contABS/ABS and Wheel torque generation/ABS Rear Right Wheel/Antilock Braking System ==
  note: Tb_LPF [Nm]
  note: Tb_Ctrl [Nm]
  note: Tb_Dr [Nm]
  note: lambda (feedback) [-]
  note: Error
  note: Tb_Ctrl [Nm]
  note: rho*Tb_LPF [Nm]
  Tb_Dr [Nm] : Inport
  lambda_ref [-] : Inport  Port=2
  lambda [-] : Inport  Port=3
  vehicle speed [m/s] : Inport  Port=4
  ABS Selection Number : Scope
  Activation and Deactivation Logic : Stateflow chart  TreatAsAtomicUnit=on
  Add2 : Sum  Inputs=+-|
  Compare To Constant : simulink/Logic and Bit Operations/Compare To Constant  relop===  const=3.0  OutDataTypeStr=boolean
  Derivative : Derivative
  Memory : Memory
  Multiport Switch : MultiPortSwitch  SaturateOnIntegerOverflow=off  InputSameDT=off
  PID Regulator : TransferFcn  Numerator=12000 * [1/400 1/10 1]  Denominator=[1/500 1 0]
  PID Regulator1 : TransferFcn  Numerator=[omega_LPF]  Denominator=[1 omega_LPF]
  Product : Product
  Sample and Hold : dspsigops/Sample and Hold  trig=Rising edge  initCond=0  latchinput=off
  Saturation1 : Saturate  UpperLimit=Tb_max  LowerLimit=0
  Scope2 : Scope
  Tb_LPF : Scope
  rho : Constant  Value=rho
  Tb [Nm] : Outport
  wires:
  lambda_ref [-]/1 -> Add2/1
  Activation and Deactivation Logic/2(ABS_ON) -> Scope2/1
  [Tb_Ctrl] -> Multiport Switch/3
  Tb_Dr [Nm]/1 -> [Tb_Driver], Derivative/1, Activation and Deactivation Logic/1(Tb_Dr)
  vehicle speed [m/s]/1 -> Activation and Deactivation Logic/3(v)
  Multiport Switch/1 -> Saturation1/1
  Add2/1 -> PID Regulator/1
  [Tb_Driver] -> Multiport Switch/2
  Derivative/1 -> Activation and Deactivation Logic/4(Tb_dot)
  lambda [-]/1 -> Activation and Deactivation Logic/6(lambda), Add2/2
  Activation and Deactivation Logic/1(Tb_select) -> ABS Selection Number/1, Multiport Switch/1, Compare To Constant/1
  Saturation1/1 -> Tb [Nm]/1
  PID Regulator/1 -> PID Regulator1/1, [Tb_Ctrl], Activation and Deactivation Logic/2(Tb_Ctrl)
  PID Regulator1/1 -> [Tb_LPF]
  [Tb_LPF] -> Sample and Hold/1
  Sample and Hold/1 -> Tb_LPF/1, Product/1, Memory/1
  Memory/1 -> Activation and Deactivation Logic/5(Tb_LPF)
  rho/1 -> Product/2
  Product/1 -> Multiport Switch/4
  Compare To Constant/1 -> Sample and Hold/Trigger

== system Vehicle_Model_contABS/Driver/Lateral Controller/Arc Path Following Controller ==
  targetPoint : Inport
  pose : Inport  Port=2
  endOfCircuit : Inport  Port=3
  Action Port : ActionPort  ActionPortLabel=case [ 1 ]:
  Arc Path Following Controller : MATLAB Function  TreatAsAtomicUnit=on
  delta : Outport  VectorParamsAs1DForOutWhenUnconnected=off
  wires:
  Arc Path Following Controller/1(delta) -> delta/1
  targetPoint/1 -> Arc Path Following Controller/1(target_Point)
  pose/1 -> Arc Path Following Controller/2(pose)
  endOfCircuit/1 -> Arc Path Following Controller/3(endOfCircuit)

== system Vehicle_Model_contABS/Driver/Lateral Controller/Lateral Controller Clothoid-based ==
  targetPoint : Inport
  pose : Inport  Port=2
  speed : Inport  Port=3
  endOfCircuit : Inport  Port=4
  Action Port : ActionPort  ActionPortLabel=case [ 4 ]:
  MATLAB System : MATLABSystem  System=clothoidBased_lateralController  lookAhead=clothoidBasedParams.lookAhead  Kus=clothoidBasedParams.Kus  L=vehicle_data.vehicle.L  SimulateUsing=Interpreted execution
      mask Type: clothoidBased_lateralController
      mask Display:
      | disp('clothoidBased_lateralController');
      | port_label('input',1,'targetPoint');
      | port_label('input',2,'vehPose');
      | port_label('input',3,'vehSpeed');
      | port_label('input',4,'endOfCircuit');
      | port_label('output',1,'delta_req');
  Selector : Selector  InputPortWidth=4  IndexOptions=Index vector (dialog)  Indices=[1 2 3]  OutputSizes=1
  delta : Outport  VectorParamsAs1DForOutWhenUnconnected=off
  wires:
  speed/1 -> MATLAB System/3
  MATLAB System/1 -> delta/1
  pose/1 -> MATLAB System/2
  targetPoint/1 -> Selector/1
  Selector/1 -> MATLAB System/1
  endOfCircuit/1 -> MATLAB System/4

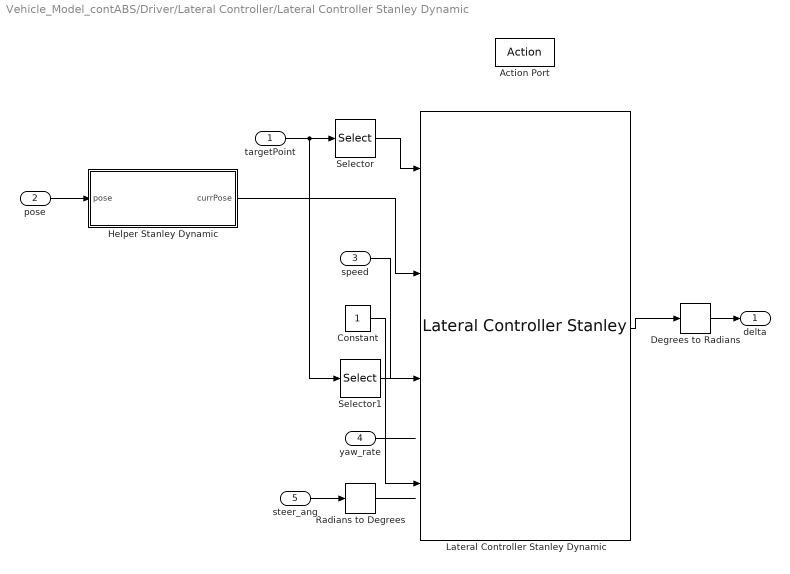
== system Vehicle_Model_contABS/Driver/Lateral Controller/Lateral Controller Stanley Dynamic ==
  targetPoint : Inport
  pose : Inport  Port=2
  speed : Inport  Port=3
  yaw_rate : Inport  Port=4
  steer_ang : Inport  Port=5
  Action Port : ActionPort  ActionPortLabel=case [ 3 ]:
  Constant : Constant
  Degrees to Radians : simulink_extras/Transformations/Degrees to Radians
  Helper Stanley Dynamic : MATLAB Function  TreatAsAtomicUnit=on
  Lateral Controller Stanley Dynamic : drivingvehiclecontroller/Lateral Controller Stanley  ModelType=Dynamic bicycle model  PositionGainF=stanleyParams.positGainFW  PositionGainR=stanleyParams.positGainREV  YawRateGain=stanleyParams.yawRateGain  DelayGain=stanleyParams.steerGain  VehicleMass=vehicle_data.vehicle.m  Lf=vehicle_data.vehicle.Lf  Lr=vehicle_data.vehicle.Lr  TireStiffness=stanleyParams.cornerStiff  Wheelbase=2.8  MaxSteeringAngle=stanleyParams.maxSteerAngle
  Radians to Degrees : simulink_extras/Transformations/Radians to Degrees
  Selector : Selector  InputPortWidth=4  IndexOptions=Index vector (dialog)  Indices=[1 2 3]  OutputSizes=1
  Selector1 : Selector  InputPortWidth=4  IndexOptions=Index vector (dialog)  Indices=[4]  OutputSizes=1
  delta : Outport  VectorParamsAs1DForOutWhenUnconnected=off
  wires:
  Lateral Controller Stanley Dynamic/1 -> Degrees to Radians/1
  pose/1 -> Helper Stanley Dynamic/1(pose)
  speed/1 -> Lateral Controller Stanley Dynamic/3
  Constant/1 -> Lateral Controller Stanley Dynamic/4
  Degrees to Radians/1 -> delta/1
  Helper Stanley Dynamic/1(currPose) -> Lateral Controller Stanley Dynamic/2
  targetPoint/1 -> Selector1/1, Selector/1
  Selector/1 -> Lateral Controller Stanley Dynamic/1
  Selector1/1 -> ?
  yaw_rate/1 -> ?
  Radians to Degrees/1 -> ?
  steer_ang/1 -> Radians to Degrees/1

== system Vehicle_Model_contABS/Driver/Lateral Controller/Lateral Controller Stanley Kinematic ==
  targetPoint : Inport
  pose : Inport  Port=2
  speed : Inport  Port=3
  Action Port : ActionPort  ActionPortLabel=case [ 2 ]:
  Constant : Constant
  Degrees to Radians : simulink_extras/Transformations/Degrees to Radians
  Helper Stanley Kinematic : MATLAB Function  TreatAsAtomicUnit=on
  Lateral Controller Stanley Kinematic : drivingvehiclecontroller/Lateral Controller Stanley  ModelType=Kinematic bicycle model  PositionGainF=stanleyParams.positGainFW  PositionGainR=stanleyParams.positGainREV  YawRateGain=0.2  DelayGain=0.2  VehicleMass=1575  Lf=1.2  Lr=1.6  TireStiffness=19000  Wheelbase=vehicle_data.vehicle.Lf + vehicle_data.vehicle.Lr  MaxSteeringAngle=stanleyParams.maxSteerAngle
  Selector : Selector  InputPortWidth=4  IndexOptions=Index vector (dialog)  Indices=[1 2 3]  OutputSizes=1
  delta : Outport  VectorParamsAs1DForOutWhenUnconnected=off
  wires:
  Lateral Controller Stanley Kinematic/1 -> Degrees to Radians/1
  pose/1 -> Helper Stanley Kinematic/1(pose)
  speed/1 -> Lateral Controller Stanley Kinematic/3
  Constant/1 -> Lateral Controller Stanley Kinematic/4
  Degrees to Radians/1 -> delta/1
  Helper Stanley Kinematic/1(currPose) -> Lateral Controller Stanley Kinematic/2
  targetPoint/1 -> Selector/1
  Selector/1 -> Lateral Controller Stanley Kinematic/1

== system Vehicle_Model_contABS/Driver/Lateral Controller/Preview point lateral Controller ==
  targetPoint : Inport
  endOfCircuit : Inport  Port=2
  Action Port : ActionPort  ActionPortLabel=case [ 5 ]:
  Constant : Constant  Value=previewPointParams.ke
  Constant1 : Constant  Value=previewPointParams.kp
  Preview Point Controller : MATLAB Function  TreatAsAtomicUnit=on
  delta : Outport  VectorParamsAs1DForOutWhenUnconnected=off
  wires:
  Preview Point Controller/1(delta) -> delta/1
  targetPoint/1 -> Preview Point Controller/1(target_Point)
  endOfCircuit/1 -> Preview Point Controller/4(endOfCircuit)
  Constant/1 -> Preview Point Controller/2(ke)
  Constant1/1 -> Preview Point Controller/3(kp)

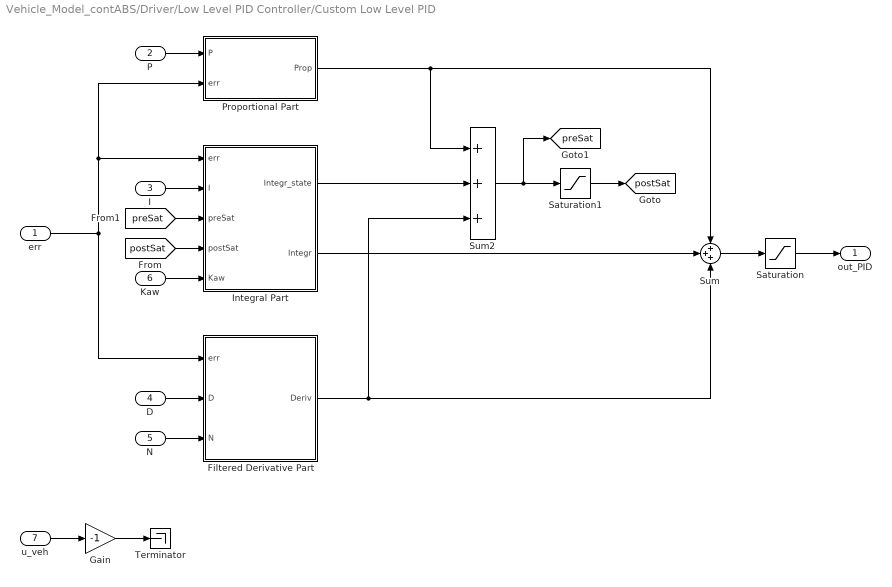
== system Vehicle_Model_contABS/Driver/Low Level PID Controller/Custom Low Level PID ==
  err : Inport
  P : Inport  Port=2
  I : Inport  Port=3
  D : Inport  Port=4
  N : Inport  Port=5
  Kaw : Inport  Port=6
  u_veh : Inport  Port=7
  Filtered Derivative Part : Subsystem
  Gain : Gain  Gain=-1
  Integral Part : Subsystem
  Proportional Part : Subsystem
  Saturation : Saturate  UpperLimit=1  LowerLimit=-1  LinearizeAsGain=off
  Saturation1 : Saturate  UpperLimit=1  LowerLimit=-1  LinearizeAsGain=off
  Sum : Sum  Inputs=+++
  Sum2 : Sum  Inputs=+++
  Terminator : Terminator
  out_PID : Outport  VectorParamsAs1DForOutWhenUnconnected=off
  tag scope: postSat=global, preSat=global
  wires:
  Sum2/1 -> [preSat], Saturation1/1
  Sum/1 -> Saturation/1
  Saturation/1 -> out_PID/1
  err/1 -> Filtered Derivative Part/1(err), Proportional Part/2(err), Integral Part/1(err)
  Saturation1/1 -> [postSat]
  I/1 -> Integral Part/2(I)
  Integral Part/1(Integr_state) -> Sum2/2
  Integral Part/2(Integr) -> Sum/2
  Proportional Part/1(Prop) -> Sum2/1, Sum/1
  P/1 -> Proportional Part/1(P)
  [preSat] -> Integral Part/3(preSat)
  [postSat] -> Integral Part/4(postSat)
  Filtered Derivative Part/1(Deriv) -> Sum/3, Sum2/3
  D/1 -> Filtered Derivative Part/2(D)
  N/1 -> Filtered Derivative Part/3(N)
  u_veh/1 -> Gain/1
  Gain/1 -> Terminator/1
  Kaw/1 -> Integral Part/5(Kaw)

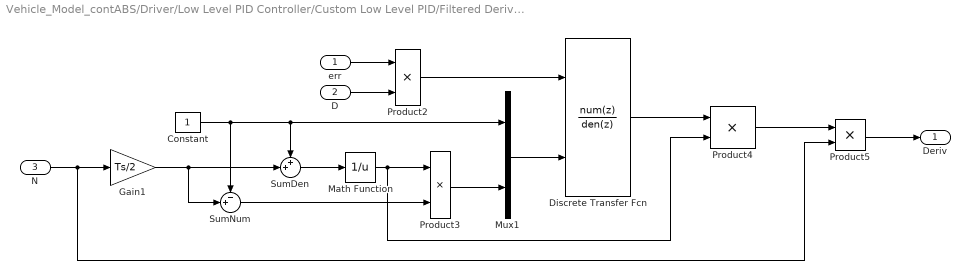
== system Vehicle_Model_contABS/Driver/Low Level PID Controller/Custom Low Level PID/Filtered Derivative Part ==
  err : Inport
  D : Inport  Port=2
  N : Inport  Port=3
  Constant : Constant
  Discrete Transfer Fcn : DiscreteTransferFcn  Numerator=[1 -1]  DenominatorSource=Input port  SampleTime=Ts  a0EqualsOne=on
      settings: InputPortMap=u0,p3
  Gain1 : Gain  Gain=Ts/2
  Math Function : Math  Operator=reciprocal  SignedPower=on
  Mux1 : Mux  Inputs=2
  Product{2..5} (4 alike) : Product
  SumDen : Sum  Inputs=++|
  SumNum : Sum  Inputs=-+|
  Deriv : Outport  VectorParamsAs1DForOutWhenUnconnected=off
  wires:
  N/1 -> Gain1/1, Product5/2
  Product4/1 -> Product5/1
  SumDen/1 -> Math Function/1
  Math Function/1 -> Product4/2, Product3/1
  SumNum/1 -> Product3/2
  Product2/1 -> Discrete Transfer Fcn/1
  Discrete Transfer Fcn/1 -> Product4/1
  Constant/1 -> SumNum/1, SumDen/1, Mux1/1
  Product3/1 -> Mux1/2
  Mux1/1 -> Discrete Transfer Fcn/2
  Gain1/1 -> SumNum/2, SumDen/2
  err/1 -> Product2/1
  D/1 -> Product2/2
  Product5/1 -> Deriv/1

== system Vehicle_Model_contABS/Driver/Low Level PID Controller/Custom Low Level PID/Integral Part ==
  err : Inport
  I : Inport  Port=2
  preSat : Inport  Port=3
  postSat : Inport  Port=4
  Kaw : Inport  Port=5
  Anti-windup : Subsystem
  Discrete-Time Integrator1 : DiscreteIntegrator  IntegratorMethod=Integration: Trapezoidal  SampleTime=Ts  ShowStatePort=on  ICPrevOutput=DiscIntNeverNeededParam  ICPrevScaledInput=DiscIntNeverNeededParam
  Product1 : Product
  Integr_state : Outport  VectorParamsAs1DForOutWhenUnconnected=off
  Integr : Outport  Port=2  VectorParamsAs1DForOutWhenUnconnected=off
  wires:
  Discrete-Time Integrator1/State -> Integr_state/1
  preSat/1 -> Anti-windup/2(preSat)
  Product1/1 -> Anti-windup/4(preInt)
  postSat/1 -> Anti-windup/3(postSat)
  I/1 -> Product1/2
  Anti-windup/1(Out_antiWindUp) -> Discrete-Time Integrator1/1
  Discrete-Time Integrator1/1 -> Integr/1
  err/1 -> Product1/1
  Kaw/1 -> Anti-windup/1(Kaw)

== system Vehicle_Model_contABS/Driver/Low Level PID Controller/Custom Low Level PID/Proportional Part ==
  P : Inport
  err : Inport  Port=2
  Product : Product
  Prop : Outport  VectorParamsAs1DForOutWhenUnconnected=off
  wires:
  P/1 -> Product/2
  Product/1 -> Prop/1
  err/1 -> Product/1

== system Vehicle_Model_contABS/Driver/Low Level PID Controller/Custom Low Level PID/Integral Part/Anti-windup ==
  Kaw : Inport
  preSat : Inport  Port=2
  postSat : Inport  Port=3
  preInt : Inport  Port=4
  Product : Product
  Sum : Sum  Inputs=|-+
  Sum1 : Sum  Inputs=|++
  Out_antiWindUp : Outport  VectorParamsAs1DForOutWhenUnconnected=off
  wires:
  preSat/1 -> Sum/1
  preInt/1 -> Sum1/2
  Product/1 -> Sum1/1
  Sum1/1 -> Out_antiWindUp/1
  Sum/1 -> Product/2
  postSat/1 -> Sum/2
  Kaw/1 -> Product/1

== matlab function Vehicle_Model_contABS/Driver/Lateral Controller/Lateral Controller Stanley Kinematic/Helper Stanley Kinematic ==
  data: pose input; currPose output
function currPose = helperStanleyKine(pose)

    currPose = [pose(1), pose(2), rad2deg(pose(3))];

end

== matlab function Vehicle_Model_contABS/ABS and Wheel torque generation/ABS Rear Right Wheel/compute lambda ==
  data: u input; lambda output; omega input; vehicle_data parameter
function lambda = compute_lambda(u, omega, vehicle_data)

lambda = (u - omega*vehicle_data.rear_wheel.Rr)/u;
